simulink model "PenduloEstabilidade"  (Simulink 7.2)
settings: Solver=ode45  StartTime=0.0  StopTime=500  RelTol=1e-3
settings Model: Creator=Leonardo  LastModifiedBy=52473520682
settings DebuggingCC: StrictBusMsg=ErrorLevel1

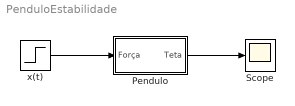
== system PenduloEstabilidade ==
  Pendulo : Subsystem
  Scope : Scope
  x(t) : Step  Time=0  After=20  SampleTime=0
  wires:
  x(t)/1 -> Pendulo/1(Força)
  Pendulo/1(Teta) -> Scope/1

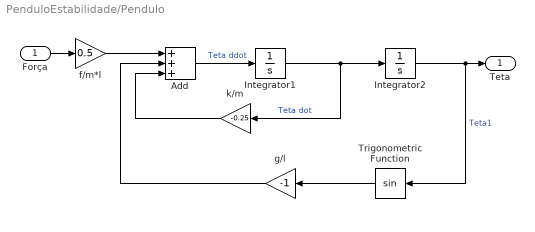
== system PenduloEstabilidade/Pendulo ==
  Força : Inport
  Add : Sum  Inputs=+++
  Integrator1 : Integrator
  Integrator2 : Integrator
  Trigonometric Function : Trigonometry  Orientation=left
  f/m*l : Gain  Gain=0.5
  g/l : Gain  Orientation=left  Gain=-1
  k/m : Gain  Orientation=left  Gain=-0.25
  Teta : Outport
  wires:
  Integrator1/1 -> Integrator2/1, k/m/1  "Teta dot"
  Add/1 -> Integrator1/1  "Teta ddot"
  Integrator2/1 -> Teta/1, Trigonometric Function/1  "Teta1"
  Trigonometric Function/1 -> g/l/1
  g/l/1 -> Add/2
  k/m/1 -> Add/3
  f/m*l/1 -> Add/1
  Força/1 -> f/m*l/1
